simulink model "Final_EWASP_VC"  (R2022a)
settings: Solver=ode1  StartTime=0.0  StopTime=24*3600  FixedStep=10  RelTol=1e-3
values from neighbouring files (symbols this model uses):
  Aux_Threshold = 52    [Setup_Code_EWASP_VC.m]
  buildingAge = 2005    [Setup_Code_EWASP_VC.m]
  ceilingHeight = 2.4    [Setup_Code_EWASP_VC.m]
  conductiveHconnectMatrix = [ ... (first row only)    [Setup_Code_EWASP_VC.m]
  cRoofGreen = 100000    [Setup_Code_EWASP_VC.m]
  Defrost_After_Time = 30    [Setup_Code_EWASP_VC.m]
  DHWDemandProfile = occFreegainHotwaterElecTestPassiveOcc3(:,3)    [Setup_Code_EWASP_VC.m]
  Elec_Max = Elec_Max*(30/24.2)    [Setup_Code_EWASP_VC.m]
  Elec_Mid = Elec_Mid*(30/24.2)    [Setup_Code_EWASP_VC.m]
  Elec_Min = Elec_Min*(30/24.2)    [Setup_Code_EWASP_VC.m]
  ElecDemandProfile = occFreegainHotwaterElecTestPassiveOcc3(:,4)    [Setup_Code_EWASP_VC.m]
  ElecFixed = [Elec_Max(6,2) Elec_Max(6,4) Elec_Max(6,6) Elec_Max(6,7) ... (first row only)    [Setup_Code_EWASP_VC.m]
  floorOrCeilingArea = floorOrCeilingArea*1.15    [Setup_Code_EWASP_VC.m]
  forceCold = 0    [Setup_Code_EWASP_VC.m]
  freegain = occFreegainHotwaterElecTestPassiveOcc3(:,2)-max(occupancy)*25    [Setup_Code_EWASP_VC.m]
  furnitureModelOn = 1    [Setup_Code_EWASP_VC.m]
  Heat_Max = Heat_Max*(30/24.2)    [Setup_Code_EWASP_VC.m]
  Heat_Mid = Heat_Mid*(30/24.2)    [Setup_Code_EWASP_VC.m]
  Heat_Min = Heat_Min*(30/24.2)    [Setup_Code_EWASP_VC.m]
  HeatFixed = [Heat_Max(6,2) Heat_Max(6,4) Heat_Max(6,6) Heat_Max(6,7) ... (first row only)    [Setup_Code_EWASP_VC.m]
  HeatingOnProfile = repmat(HeatingOnProfile,365,1)    [Setup_Code_EWASP_VC.m]
  HEX_ReturnLowerLimit = 52.5    [Setup_Code_EWASP_VC.m]
  HEX_ReturnUpperLimit = 55    [Setup_Code_EWASP_VC.m]
  LeakMultiplier = 1+(2*(rand()-0.5)/10)    [Setup_Code_EWASP_VC.m]
  loopCap = 15    [Setup_Code_EWASP_VC.m]
  maxOcc = max(occupancyProfile)    [Setup_Code_EWASP_VC.m]
  NESW_wallArea = max(NESW_Lengths*ceilingHeight-NESW_Windows,0)    [Setup_Code_EWASP_VC.m]
  NESW_Windows = [ ... (first row only)    [Setup_Code_EWASP_VC.m]
  numRooms = roomCount    [Setup_Code_EWASP_VC.m]
  offsetDays = 0    [Setup_Code_EWASP_VC.m]
  pumpChoice = pumpChoices(MinIndex,1)    [Setup_Code_EWASP_VC.m]
  pumpRamp = 180    [Setup_Code_EWASP_VC.m]
  ReturnLowerLimit = 37.5    [Setup_Code_EWASP_VC.m]
  ReturnUpperLimit = 40    [Setup_Code_EWASP_VC.m]
  RoofIrradiance = Flat_NS_EW_RoofIrradiance(:,1)    [Setup_Code_EWASP_VC.m]
  roofStartTemp = ones(11,1)*20    [Setup_Code_EWASP_VC.m]
  rooftype = 0    [Setup_Code_EWASP_VC.m]
  RoomDataMatrix = [zeros(1,12);ones(1,12)*wallDensity;zeros(1,12);ones(1,12)*wallU;ones(1,12)*windowU;ones(1,12)*floorU;ones(1,12)*ceilingU;zeros(1,12);windowArea, 0;floorOrCeilingArea;zeros(1,12);floorOrCeilingArea*ceilingHeight]    [Setup_Code_EWASP_VC.m]
  roomVol = roomVol*1.15    [Setup_Code_EWASP_VC.m]
  slabStartTemp = (GroundTempTimeSeries(offsetDays*1440+1,1)+thermostatSetting)/2    [Setup_Code_EWASP_VC.m]
  SlackRequest = zeros(1440,1)    [Setup_Code_EWASP_VC.m]
  SolarThermalExists = 0    [Setup_Code_EWASP_VC.m]
  SourceFixed = HeatFixed-ElecFixed    [Setup_Code_EWASP_VC.m]
  StateSeries = StateSeriesGenerator(22,7,1)    [Setup_Code_EWASP_VC.m]
  Tank_Lower_Temp = 49.5    [Setup_Code_EWASP_VC.m]
  Tank_Upper_Temp = 52    [Setup_Code_EWASP_VC.m]
  Tank_Volume_m3 = 0.15    [Setup_Code_EWASP_VC.m]
  TankHeatHour = randi([1 5])-1    [Setup_Code_EWASP_VC.m]
  thermostatSetting = 20.0    (= 20)    [Setup_Code_EWASP_VC.m]
  upDown = [0;0;0;0;1;1;1;1;1;1;1]    [Setup_Code_EWASP_VC.m]
  variableASHP = 1    [Setup_Code_EWASP_VC.m]
  wallStartTempExt = thermostatSetting*(0.266+0.00215*outdoorStartTemp+0.018*wallU+0.00113*outdoorStartTemp*wallU+0.0068*wallU^2)    [Setup_Code_EWASP_VC.m]
undefined symbols (not defined in the file or in its folder): a, ceilingU, condUDMatrix, convUDMatrix, deltaPEXPANDED_E, deltaPEXPANDED_E2, deltaPEXPANDED_N, deltaPEXPANDED_N2, deltaPEXPANDED_S, deltaPEXPANDED_S2, deltaPEXPANDED_W, deltaPEXPANDED_W2, DesiredDHWTemp, DesiredFlowTempVsInOutDeltaTemp, DiffuseHorizontal, DiscIntNeverNeededParam, DNI, dwnAndConcrete, DWORK_A_HX, DWORK_CHK_FLU, DWORK_CP_NODE, DWORK_DH, DWORK_FLUID, DWORK_HCON, DWORK_LOSS, DWORK_MDOTDOWN, DWORK_MDOTIN, DWORK_MDOTUP, DWORK_MIX, DWORK_PRESS, DWORK_QDOTIN, DWORK_RHO_NODE, DWORK_TIN, DWORK_TS_OLD, DWORK_V_NODE, GroundTempTimeSeries, HCM, HCM2, HCM_closed, HCM_closed2, intermediateU, IsTop, massFlowMatrix, neighbourMatrix, numericalRoomUse, RadiatorMatrix, room2roomflowmatrix_E, room2roomflowmatrix_E2, room2roomflowmatrix_N, room2roomflowmatrix_N2, room2roomflowmatrix_S, room2roomflowmatrix_S2, room2roomflowmatrix_W, room2roomflowmatrix_W2, StateAirInEXPANDED_E, StateAirInEXPANDED_E2, StateAirInEXPANDED_N, StateAirInEXPANDED_N2, StateAirInEXPANDED_S, StateAirInEXPANDED_S2 ... (+23)
libraries: simulink x6, dspsigops x4, dspmtrx3 x4, carnot x3, spsEdgeDetectorLib x2, dspstat3 x2, powerlib_meascontrol x1, simulink_extras x1
(part 13 of 27)

== system Final_EWASP_VC/Airflow Model/Subsystem1/Subsystem ==
  In1 : Inport
  In2 : Inport  Port=2
  In3 : Inport  Port=3
  In4 : Inport  Port=4
  In5 : Inport  Port=5
  In6 : Inport  Port=6
  Abs{1..4,6} (5 alike) : Abs  SaturateOnIntegerOverflow=off
  Absolute Heat From : Product  Inputs=3
  Absolute Heat In2 : Product  Inputs=3
  Absolute Heat Out : Product  Inputs=3
  Absolute Heat Out1 : Product  Inputs=3
  Actual buoyancy : MATLAB Function  TreatAsAtomicUnit=on
  Add : Sum  Inputs=4
  Add1 : Sum  Inputs=4
  Add2 : Sum  Inputs=+-
  Air Heat capacity{,1..3} (4 alike) : Constant  Value=1000
  Celcius to Kelvin{,1,4..5} (4 alike) : Constant  Value=273.15
  "Determine flow in and flow out from net flow (+ve out, -ve in)" : Subsystem
  "Net flow out of room to neighbouring room (+ve out, -ve in)1" : Constant  Value=HCM_closed
  "Net flow out of room to neighbouring room (+ve out, -ve in)3" : Constant  Value=HCM
  "Net flow out of room to neighbouring room (+ve out, -ve in)5" : Constant  Value=VCM
  Product1 : Product
  Remove nan values : MATLAB Function  TreatAsAtomicUnit=on
  Saturation : Saturate  UpperLimit=100  LowerLimit=0
  Saturation1 : Saturate  UpperLimit=0  LowerLimit=-100
  Saturation2 : Saturate  UpperLimit=100  LowerLimit=0
  Saturation3 : Saturate  UpperLimit=0  LowerLimit=-100
  Subsystem : Subsystem
  Subsystem1 : Subsystem
      mask Display:
      | port_label('output', 1, 'Average_Density_Matrix')
      | port_label('output', 2, 'Delta_Density_Matrix')
      | port_label('input', 1, 'Room_Temp_Vector')
  Sum{,1,3..4} (4 alike) : Sum  Inputs=|++
  Sum of Elements : Sum  Inputs=+  CollapseMode=Specified dimension  CollapseDim=2
  Sum of Elements1 : Sum  Inputs=+  CollapseMode=Specified dimension  CollapseDim=2
  Sum2 : Sum  Inputs=+-
  Sum5 : Sum  Inputs=-++
  Sum6 : Sum  Inputs=+-
  max buoyancy : MATLAB Function  TreatAsAtomicUnit=on
  pflood : MATLAB Function  TreatAsAtomicUnit=on
  remove data no related to vertical flow : Constant  Value=VCM
  remove verical forced and closed door flow from bidirectinality calc1 : Product
  remove verical forced and closed door flow from bidirectinality calc2 : Product
  remove verical forced and closed door flow from bidirectinality calc : Product
  setnegative buoyancy flow to zero : Saturate  UpperLimit=100  LowerLimit=0
  tempVector to matrices : MATLAB Function  TreatAsAtomicUnit=on
  Out1 : Outport  VectorParamsAs1DForOutWhenUnconnected=off
  wires:
  [SAI] -> Absolute Heat In2/1
  [closed_out] -> Add1/2
  [open_out] -> Add1/1
  [R2R] -> remove verical forced and closed door flow from bidirectinality calc1/2, remove verical forced and closed door flow from bidirectinality calc/2
  remove data no related to vertical flow/1 -> Abs3/1
  "Net flow out of room to neighbouring room (+ve out, -ve in)1"/1 -> remove verical forced and closed door flow from bidirectinality calc1/1
  Sum1/1 -> Absolute Heat From/2
  Product1/1 -> Remove nan values/1(u)
  Saturation1/1 -> Abs1/1
  Abs3/1 -> Product1/2
  "Net flow out of room to neighbouring room (+ve out, -ve in)3"/1 -> remove verical forced and closed door flow from bidirectinality calc/1
  tempVector to matrices/1(y) -> [roomTempMatrix]
  setnegative buoyancy flow to zero/1 -> Product1/1
  remove verical forced and closed door flow from bidirectinality calc/1 -> "Determine flow in and flow out from net flow (+ve out, -ve in)"/1(In1)
  In6/1 -> [ODT]
  max buoyancy/1(y) -> Actual buoyancy/3(w)
  "Net flow out of room to neighbouring room (+ve out, -ve in)5"/1 -> Abs4/1
  Sum4/1 -> Absolute Heat In2/2
  Remove nan values/1(y) -> [buoyancy_in], [buoyancy_out]
  Sum of Elements1/1 -> Sum2/2
  Air Heat capacity/1 -> Absolute Heat Out/3
  Sum5/1 -> Out1/1
  Abs4/1 -> remove verical forced and closed door flow from bidirectinality calc2/2
  "Determine flow in and flow out from net flow (+ve out, -ve in)"/2(Out2) -> Subsystem/2(In2)
  remove verical forced and closed door flow from bidirectinality calc1/1 -> Saturation/1, Saturation1/1
  Add/1 -> Absolute Heat From/1, Add2/1
  Absolute Heat Out/1 -> Sum of Elements1/1
  Absolute Heat From/1 -> Sum of Elements/1
  Sum/1 -> Absolute Heat Out/2
  pflood/1(y) -> Abs2/1
  Saturation3/1 -> Abs6/1
  Abs6/1 -> [vforce_in]
  Saturation2/1 -> [vforce_out]
  Saturation/1 -> [closed_out]
  Add1/1 -> Add2/2, Absolute Heat Out/1
  Subsystem1/2(Out2) -> pflood/1(u)
  Absolute Heat In2/1 -> Sum5/3
  [TVT] -> Subsystem1/1(In1)
  remove verical forced and closed door flow from bidirectinality calc2/1 -> Saturation2/1, Saturation3/1
  [DP] -> Actual buoyancy/1(u)
  Sum2/1 -> Sum5/2
  [neighTempMatrix] -> Sum1/1
  [roomTempMatrix] -> Sum6/1
  Subsystem1/1(Out1) -> max buoyancy/1(u)
  Actual buoyancy/1(y) -> setnegative buoyancy flow to zero/1
  Abs2/1 -> Actual buoyancy/2(v), max buoyancy/2(v)
  [roomTempMatrix] -> Sum/1
  [SAO] -> Absolute Heat Out1/2
  Abs1/1 -> [closed_in]
  [neighTempMatrix] -> Sum6/2
  [R2R] -> remove verical forced and closed door flow from bidirectinality calc2/1
  Celcius to Kelvin5/1 -> Sum4/2
  Air Heat capacity3/1 -> Absolute Heat In2/3
  [TVT] -> tempVector to matrices/1(u)
  Celcius to Kelvin4/1 -> Sum3/2
  Air Heat capacity2/1 -> Absolute Heat Out1/3
  Celcius to Kelvin1/1 -> Sum1/2
  Air Heat capacity1/1 -> Absolute Heat From/3
  [TVT] -> Sum3/1
  tempVector to matrices/2(x) -> [neighTempMatrix]
  [ODT] -> Sum4/1
  In5/1 -> [TVT]
  Sum6/1 -> "Determine flow in and flow out from net flow (+ve out, -ve in)"/2(In2)
  [open_in] -> Add/1
  [closed_in] -> Add/2
  Celcius to Kelvin/1 -> Sum/2
  In2/1 -> [DP]
  In1/1 -> [R2R]
  In3/1 -> [SAO]
  In4/1 -> [SAI]
  Absolute Heat Out1/1 -> Sum5/1
  Sum3/1 -> Absolute Heat Out1/1
  Sum of Elements/1 -> Sum2/1
  "Determine flow in and flow out from net flow (+ve out, -ve in)"/1(Out1) -> Subsystem/1(In1)
  Subsystem/1(Out1) -> [open_in]
  Subsystem/2(Out2) -> [open_out]
  [vforce_in] -> Add/4
  [vforce_out] -> Add1/4
  [buoyancy_in] -> Add/3
  [buoyancy_out] -> Add1/3

== system Final_EWASP_VC/Airflow Model/Subsystem2/Subsystem ==
  In1 : Inport
  In2 : Inport  Port=2
  In3 : Inport  Port=3
  In4 : Inport  Port=4
  In5 : Inport  Port=5
  In6 : Inport  Port=6
  Abs{1..4,6} (5 alike) : Abs  SaturateOnIntegerOverflow=off
  Absolute Heat From : Product  Inputs=3
  Absolute Heat In2 : Product  Inputs=3
  Absolute Heat Out : Product  Inputs=3
  Absolute Heat Out1 : Product  Inputs=3
  Actual buoyancy : MATLAB Function  TreatAsAtomicUnit=on
  Add : Sum  Inputs=4
  Add1 : Sum  Inputs=4
  Air Heat capacity{,1..3} (4 alike) : Constant  Value=1000
  Celcius to Kelvin{,1,4..5} (4 alike) : Constant  Value=273.15
  "Determine flow in and flow out from net flow (+ve out, -ve in)" : Subsystem  TreatAsAtomicUnit=on
  "Net flow out of room to neighbouring room (+ve out, -ve in)1" : Constant  Value=HCM_closed2
  "Net flow out of room to neighbouring room (+ve out, -ve in)3" : Constant  Value=HCM2
  "Net flow out of room to neighbouring room (+ve out, -ve in)5" : Constant  Value=VCM2
  Product1 : Product
  Remove nan values : MATLAB Function  TreatAsAtomicUnit=on
  Saturation : Saturate  UpperLimit=100  LowerLimit=0
  Saturation1 : Saturate  UpperLimit=0  LowerLimit=-100
  Saturation2 : Saturate  UpperLimit=100  LowerLimit=0
  Saturation3 : Saturate  UpperLimit=0  LowerLimit=-100
  Subsystem1 : Subsystem
      mask Display:
      | port_label('output', 1, 'Average_Density_Matrix')
      | port_label('output', 2, 'Delta_Density_Matrix')
      | port_label('input', 1, 'Room_Temp_Vector')
  Sum{,1,3..4} (4 alike) : Sum  Inputs=|++
  Sum of Elements : Sum  Inputs=+  CollapseMode=Specified dimension  CollapseDim=2
  Sum of Elements1 : Sum  Inputs=+  CollapseMode=Specified dimension  CollapseDim=2
  Sum2 : Sum  Inputs=+-
  Sum5 : Sum  Inputs=-++
  Sum6 : Sum  Inputs=+-
  Sum7 : Sum  Inputs=|-+
  Symmetry Mod : Subsystem
  max buoyancy : MATLAB Function  TreatAsAtomicUnit=on
  pflood : MATLAB Function  TreatAsAtomicUnit=on
  remove data no related to vertical flow : Constant  Value=VCM2
  remove verical forced and closed door flow from bidirectinality calc1 : Product
  remove verical forced and closed door flow from bidirectinality calc2 : Product
  remove verical forced and closed door flow from bidirectinality calc : Product
  setnegative buoyancy flow to zero : Saturate  UpperLimit=100  LowerLimit=0
  tempVector to matrices : MATLAB Function  TreatAsAtomicUnit=on
  Out1 : Outport  VectorParamsAs1DForOutWhenUnconnected=off
  wires:
  [SAI] -> Absolute Heat In2/1
  [closed_out] -> Add1/2
  [open_out] -> Add1/1
  [R2R] -> remove verical forced and closed door flow from bidirectinality calc1/2, remove verical forced and closed door flow from bidirectinality calc/2
  remove data no related to vertical flow/1 -> Abs3/1
  "Net flow out of room to neighbouring room (+ve out, -ve in)1"/1 -> remove verical forced and closed door flow from bidirectinality calc1/1
  Sum1/1 -> Absolute Heat From/2
  Product1/1 -> Remove nan values/1(u)
  Saturation1/1 -> Abs1/1
  Abs3/1 -> Product1/2
  "Net flow out of room to neighbouring room (+ve out, -ve in)3"/1 -> remove verical forced and closed door flow from bidirectinality calc/1
  tempVector to matrices/1(y) -> [roomTempMatrix]
  setnegative buoyancy flow to zero/1 -> Product1/1
  remove verical forced and closed door flow from bidirectinality calc/1 -> "Determine flow in and flow out from net flow (+ve out, -ve in)"/1(In1)
  In6/1 -> [ODT]
  max buoyancy/1(y) -> Actual buoyancy/3(w)
  "Net flow out of room to neighbouring room (+ve out, -ve in)5"/1 -> Abs4/1
  Sum4/1 -> Absolute Heat In2/2
  Remove nan values/1(y) -> [buoyancy_in], [buoyancy_out]
  Air Heat capacity/1 -> Absolute Heat Out/3
  Sum5/1 -> Out1/1
  Abs4/1 -> remove verical forced and closed door flow from bidirectinality calc2/2
  remove verical forced and closed door flow from bidirectinality calc1/1 -> Saturation/1, Saturation1/1
  Sum/1 -> Absolute Heat Out/2
  pflood/1(y) -> Abs2/1
  [buoyancy_in] -> Add/3
  Saturation3/1 -> Abs6/1
  Abs6/1 -> [vforce_in]
  [vforce_out] -> Add1/4
  Saturation2/1 -> [vforce_out]
  Absolute Heat Out1/1 -> Sum7/1, Sum5/1
  Add1/1 -> Absolute Heat Out/1
  Subsystem1/2(Out2) -> pflood/1(u)
  Absolute Heat In2/1 -> Sum7/2, Sum5/3
  [TVT] -> Subsystem1/1(In1)
  remove verical forced and closed door flow from bidirectinality calc2/1 -> Saturation2/1, Saturation3/1
  "Determine flow in and flow out from net flow (+ve out, -ve in)"/1(Out1) -> Symmetry Mod/1(In1)
  [DP] -> Actual buoyancy/1(u)
  Sum2/1 -> Sum5/2
  [neighTempMatrix] -> Sum1/1
  [roomTempMatrix] -> Sum6/1
  Subsystem1/1(Out1) -> max buoyancy/1(u)
  Actual buoyancy/1(y) -> setnegative buoyancy flow to zero/1
  Abs2/1 -> Actual buoyancy/2(v), max buoyancy/2(v)
  [roomTempMatrix] -> Sum/1
  [SAO] -> Absolute Heat Out1/2
  [vforce_in] -> Add/4
  Abs1/1 -> [closed_in]
  [neighTempMatrix] -> Sum6/2
  [R2R] -> remove verical forced and closed door flow from bidirectinality calc2/1
  Celcius to Kelvin5/1 -> Sum4/2
  Air Heat capacity3/1 -> Absolute Heat In2/3
  [TVT] -> tempVector to matrices/1(u)
  Celcius to Kelvin4/1 -> Sum3/2
  Air Heat capacity2/1 -> Absolute Heat Out1/3
  Celcius to Kelvin1/1 -> Sum1/2
  Air Heat capacity1/1 -> Absolute Heat From/3
  [TVT] -> Sum3/1
  tempVector to matrices/2(x) -> [neighTempMatrix]
  Sum3/1 -> Absolute Heat Out1/1
  [ODT] -> Sum4/1
  In5/1 -> [TVT]
  Sum6/1 -> "Determine flow in and flow out from net flow (+ve out, -ve in)"/2(In2)
  [open_in] -> Add/1
  [closed_in] -> Add/2
  Celcius to Kelvin/1 -> Sum/2
  In2/1 -> [DP]
  In1/1 -> [R2R]
  In3/1 -> [SAO]
  In4/1 -> [SAI]
  Add/1 -> Absolute Heat From/1
  Sum of Elements/1 -> Sum2/1
  Sum of Elements1/1 -> Sum2/2
  Saturation/1 -> [closed_out]
  [buoyancy_out] -> Add1/3
  Absolute Heat From/1 -> Sum of Elements/1
  Absolute Heat Out/1 -> Sum of Elements1/1
  "Determine flow in and flow out from net flow (+ve out, -ve in)"/2(Out2) -> Symmetry Mod/2(In2)
  Symmetry Mod/1(Out1) -> [open_in]
  Symmetry Mod/2(Out2) -> [open_out]

== system Final_EWASP_VC/GSHP_Subsystem/DHW for GSHP case/HeatPump_Simplified ==
  THBsource : Inport
  THB_r : Inport  Port=2
  Tamb : Inport  Port=3
  Ctrl : Inport  Port=4
  mdot_cold : Inport  Port=5
  mdot_hot : Inport  Port=6
  HeatPump_basic : Subsystem  AncestorBlock=carnot/Basic/Thermal_Models/HeatPump_basic  mask(heat pump){K=K, caph=caph, capc=capc, UA=UA}
      mask prompts: K "Parameters K (see also HP_param.m)"; caph "thermal capacity hot loop [J/K]"; capc "thermal capacity cold loop [J/K]"; UA "heat loss coefficient [W/K]"
      mask help:
      | Linearized heat pump model, uses measured data according to EN 14511 as input (Schwamberger, K.: Fortschrittsberichete VDI, Nr. 263, 1991).
      | heating power: Qdot_h = K1*Tcold_in + K2*Thot_out + K3
      | electric power: Pel = K4*Tcold_in + K5*Thot_out + K6
      | source power: Qdot_c = -K7*Tcold_in - K8*Thot_out - K9
      | differential equation: cap*dTh/dt = Qdot + mdot*cp*(T_in-T) + UA*(Tamb-T)
      | with: cap = mass * heat_capactiy
      | See hp_param.m for the parameters K1 to K9.
      mask Help: web(fullfile(path_carnot('help'),'HeatPump_basic.html'),'-helpbrowser')
      mask DialogControl ParameterTabVar0 Prompt: HP Caracteristic
      mask DialogControl ParameterTabVar01 Prompt: Thermal
      mask Display: plot(0,-30,120,130,[30,46,36,46,36,46,30],[40,40,50,60,70,80,80],[70,54,64,54,64,54,64,54,64,54,70],[40,40,44,50,55,60,65,70,75,80,80],[56,45],[95,95],[51,51],[82,95])
  T_source : Outport  VectorParamsAs1DForOutWhenUnconnected=off
  "T_out " : Outport  Port=2  VectorParamsAs1DForOutWhenUnconnected=off
  HPdat : Outport  Port=3  VectorParamsAs1DForOutWhenUnconnected=off
  Real P_Therm : Outport  Port=4  VectorParamsAs1DForOutWhenUnconnected=off
  wires:
  HeatPump_basic/2(THBload) -> "T_out "/1  "THB_s"
  THBsource/1 -> HeatPump_basic/1(Tin_cold)
  THB_r/1 -> HeatPump_basic/2(Tin_hot)
  Tamb/1 -> HeatPump_basic/3(Tamb)
  Ctrl/1 -> HeatPump_basic/4(Ctrl)
  HeatPump_basic/1(Tsource) -> T_source/1  "THBsource"
  HeatPump_basic/3(HPdat) -> HPdat/1
  HeatPump_basic/4(Real P_Therm) -> Real P_Therm/1
  mdot_cold/1 -> HeatPump_basic/5(mdot_in_cold)
  mdot_hot/1 -> HeatPump_basic/6(mdot_in_hot)

== system Final_EWASP_VC/GSHP_Subsystem/DHW for GSHP case/Storage_Type_2_CONF ==
  note: upper heat exchanger (backup heater)
  note: pipe connection for DHW
  note: pipe connection for DHW circulation
  Tamb : Inport
  Temp_HX : Inport  Port=2
  THB_dhw : Inport  Port=3
  THB_circ : Inport  Port=4
  Mdot_dhw1 : Inport  Port=5
  Mdot_dhw2 : Inport  Port=6
  mdotHEX : Inport  Port=7
  HX_EN12977_1 : Subsystem  AncestorBlock=carnot/Storage/Thermal/Storage_Ports/HX_EN12977  mask(heat exchanger for storage, data EN 12977){h_in=hx1inlet, h_out=hx1outlet, hgt=hgt, dia=hx1dia, height=-0.68756, ua0=hx1uac, uam=hx1uam, uat=hx1uat, dpqua=hx1dpqua, nodes=nodes}
      mask prompts: h_in "relative height of inlet"; h_out "relative height of outlet"; hgt "Height of storage in m"; dia "Diameter of HX pipe [m]"; height "Height difference inlet-outlet [m]"; ua0 "uac: heat transfer coefficient [W/K /(kg/s) /(°C)]"; uam "uam: massflow dependent heat transfer [-]"; uat "uat: temperature difference dependent heat transfer [-]"; dpqua "Pressure drop coefficient dpqua [Pa/(kg/s)²]"; nodes "number of nodes"
      mask help:
      | The block transforms the incoming THV vector to a vector which the storage interprets as a heat exchanger.
      | Give inlet and outlet as a relative position 0=bottom to 1=top
      | The heat transfer is calculated by:
      | UA = uac * mdot^uam * ((Theatexchanger+Tstorage)/2)^uat
      mask init: same as Final_EWASP_VC/ASHP_Subsystem/DHW for ASHP Case/Storage_Type_2_CONF/HX_EN12977_1
      mask Help: web(['file:///' fullfile(path_carnot('help'),'StoragePorts_HeatExchangerModels.html')],'-helpbrowser')
      mask TypeOptions dia: Pressure_Drop_StorageHX/dia
      mask TypeOptions height: Pressure_Drop_StorageHX/hgt
      mask TypeOptions ua0: sfun_storage_heatexchanger/p1
      mask TypeOptions uam: sfun_storage_heatexchanger/p2
      mask TypeOptions uat: sfun_storage_heatexchanger/p3
      mask TypeOptions dpqua: Pressure_Drop_StorageHX/dpqua
      mask TypeOptions nodes: sfun_storage_heatexchanger/nodes
      mask DialogControl ParameterTabVar0 Prompt: Geometry
      mask DialogControl ParameterTabVar01 Prompt: Heat transfer
      mask DialogControl ParameterTabVar012 Prompt: Pressure drop
      mask DialogControl ParameterTabVar0123 Prompt: Calculation
      mask Display: disp('HX EN12977')
  Mux : Mux  Inputs=2
  Mux1 : Mux  Inputs=2
  Pipe_Connection_1 : Subsystem  AncestorBlock=carnot/Storage/Thermal/Storage_Ports/Pipe_Connection  mask(pipe connection to storage){h_in=pipe1inlet, h_out=pipe1outlet, hgt=hgt, nodes=nodes}
      mask prompts: h_in "relative height of inlet, range from 0 (= bottom) to 1 (= top)"; h_out "relative height of outlet, range from 0 (= bottom) to 1 (= top)"; hgt "Height of storage in m"; nodes "Number of nodes of storage (DO NOT CHANGE)"
      mask help: The block transforms the incoming THV vector to a vector which the storage interprets as a flow into the storage fluid.
      mask init: same as Final_EWASP_VC/ASHP_Subsystem/DHW for ASHP Case/Storage_Type_2_CONF/Pipe_Connection_1
      mask Help: web(fullfile(path_carnot('help'),'StoragePorts_PipeConnections.html'),'-helpbrowser')
      mask DialogControl ParameterTabVar0 Prompt: Geometry
      mask DialogControl ParameterTabVar02 Prompt: Calulation
      mask Display: disp('Pipe')
  Pipe_Connection_2 : Subsystem  AncestorBlock=carnot/Storage/Thermal/Storage_Ports/Pipe_Connection  mask(pipe connection to storage){h_in=pipe2inlet, h_out=pipe2outlet, hgt=hgt, nodes=nodes}
      mask prompts: h_in "relative height of inlet, range from 0 (= bottom) to 1 (= top)"; h_out "relative height of outlet, range from 0 (= bottom) to 1 (= top)"; hgt "Height of storage in m"; nodes "Number of nodes of storage (DO NOT CHANGE)"
      mask help: The block transforms the incoming THV vector to a vector which the storage interprets as a flow into the storage fluid.
      mask init: same as Final_EWASP_VC/ASHP_Subsystem/DHW for ASHP Case/Storage_Type_2_CONF/Pipe_Connection_1
      mask Help: web(fullfile(path_carnot('help'),'StoragePorts_PipeConnections.html'),'-helpbrowser')
      mask DialogControl ParameterTabVar0 Prompt: Geometry
      mask DialogControl ParameterTabVar02 Prompt: Calulation
      mask Display: disp('Pipe')
  Scope : Scope
  Scope1 : Scope
  Scope2 : Scope
  T_Sensor_Surface : carnot/Control/T_Sensor_Surface  pos=Tsensor  tdel=10  t0=mean(tini)
      settings: SourceProductName=Carnot
  Terminator1 : Terminator
  sfun_storageTnodesjh : S-Function  AncestorBlock=carnot/Basic/Thermal_Models/sfun_storageTnodes  FunctionName=storage_TnodesMOD  Parameters=dia, volume, standing, uloss , ubot, utop, cond, tini, nodes, nconnect, elimthermocline, condinvtc  SFunctionDeploymentMode=off  EnableBusSupport=off  SFcnStateName=DWORK_DH  mask(sfunction storage_Tnodes){uloss=uwall, ubot=ubot, utop=utop, cond=axcond, volume=volume, dia=dia, standing=standing cylinder, tini=tini, nodes=nodes, nconnect=3, elimthermocline=1, condinvtc=1e5}
      mask prompts: uloss "Heat transfer coefficient to ambient [W/m²K]"; ubot "Heat transfer coefficient to ambient bottom [W/m²K]"; utop "Heat transfer coefficient to ambient top [W/m²K]"; cond "Effective thermal conductivity [W/m/K]"; volume "Volume [m³]"; dia "Diameter [m]"; standing "Position"; tini "Initial temperature in °C"; nodes "Number of nodes"; nconnect "Number of ports"; elimthermocline "Elimination method (0 = off, 1 = temperature dependant, 2 = density dependant)"; condinvtc "COND_ITC: heat transport coefficient for the method 2"
      mask help:
      | The differential equation is derived from the energy conservation equation by using the finite volume method [Patankar: Numerical Heat Transfer and Fluid Flow, 1980].
      | Methods to eliminate the inversed thermocline (It occurs when node with lower density is below a node with higher density. Typically it can be translated to a node with higher temperature below a node with lower temperature. Exception is water below 4°C.):
      | 0 - inversed thermocline is not eliminated
      | 1 - Temperature based: An inversed thermocline exists , if the  temperature of the lower node is more than LIMIT_T_INVERSED degrees  above the upper node. In that case the temperatures of the nodes are mixed. For the geometry of a laying cylinder the different volumes of the nodes are taken in account.
      |  2 - Density based : An inversed thermocline exists, if the density of the lower node is less than the density of the upper node. The model  adds an additional heat transport towards the upper node:
      | heat transport [W/m³] = COND_ITC[W*m³/kg] * density_differnce[kg/m³] / node[m³]
      mask init: same as Final_EWASP_VC/ASHP_Subsystem/DHW for ASHP Case/Storage_Type_2_CONF/sfun_storageTnodesjh
      settings: SFcnIsStateOwnerBlock=on
      mask Help: web(fullfile(path_carnot('help'),'Storage_Type_N.html'),'-helpbrowser')
      mask TypeOptions standing: standing cylinder | lying cylinder
      mask DialogControl Container5 Prompt: Thermal
      mask DialogControl Container6 Prompt: Geometry
      mask DialogControl Container7 Prompt: Caclulation
      mask DialogControl Container10 Prompt: Inversed thermocline
      mask Display:
      | disp('storage_Tnodes')
      | 
      | port_label('input', 1, 'Tamb')
      | port_label('output', 1, 'Energy')
      | port_label('output', 2, 'Tnodes')
      | 
      | if exist('nconnect','var')
      |     for n = 1:nconnect
      |         port_label('input',  n+1, ['port' num2str(n)])
      |     end
      | end
  Tsensors : Outport  VectorParamsAs1DForOutWhenUnconnected=off
  THB_hx : Outport  Port=2  VectorParamsAs1DForOutWhenUnconnected=off
  THBdhw : Outport  Port=3  VectorParamsAs1DForOutWhenUnconnected=off
  AuxHeat : Outport  Port=4  VectorParamsAs1DForOutWhenUnconnected=off
  wires:
  HX_EN12977_1/1(to_storeT) -> sfun_storageTnodesjh/4
  Pipe_Connection_2/1(to_storeT) -> Scope/1, sfun_storageTnodesjh/3
  THB_circ/1 -> Mux1/1  "THBinPipe2"
  Tamb/1 -> sfun_storageTnodesjh/1  "Tamb"
  sfun_storageTnodesjh/2 -> Scope2/1, T_Sensor_Surface/1, HX_EN12977_1/1(from_storeT)  "Tnodes"
  Pipe_Connection_1/1(to_storeT) -> THBdhw/1, sfun_storageTnodesjh/2, Scope1/1
  Temp_HX/1 -> HX_EN12977_1/2(Tempin)
  HX_EN12977_1/2(TempHEXout) -> THB_hx/1
  T_Sensor_Surface/1 -> Tsensors/1
  Mdot_dhw1/1 -> Mux/2  "THBinPipe1"
  sfun_storageTnodesjh/1 -> Terminator1/1  "Energy"
  Mdot_dhw2/1 -> Mux1/2  "THBinPipe1"
  THB_dhw/1 -> Mux/1  "THBinPipe1"
  Mux/1 -> Pipe_Connection_1/1(THBin)
  Mux1/1 -> Pipe_Connection_2/1(THBin)
  mdotHEX/1 -> HX_EN12977_1/3(massFlowIn)
  HX_EN12977_1/3(AuxHeat) -> AuxHeat/1

== system Final_EWASP_VC/GSHP_Subsystem/DHW for GSHP case/Subsystem ==
  In1 : Inport
  Ceil : Rounding
  Clock : Clock
  Constant1 : Constant  Value=60
  Constant2 : Constant  Value=60
  Direct Lookup Table (n-D) : LookupNDDirect  NumberOfTableDimensions=1  TableIsInput=on
  Divide : Product  Inputs=*/
  Divide1 : Product  Inputs=*/
  Saturation : Saturate  UpperLimit=1440*365  LowerLimit=0
  Scope : Scope
  Out1 : Outport  VectorParamsAs1DForOutWhenUnconnected=off
  wires:
  Saturation/1 -> Scope/1, Direct Lookup Table (n-D)/1
  Divide1/1 -> Direct Lookup Table (n-D)/2
  Divide/1 -> Ceil/1
  Constant1/1 -> Divide/2
  In1/1 -> Divide1/1
  Direct Lookup Table (n-D)/1 -> Out1/1
  Constant2/1 -> Divide1/2
  Clock/1 -> Divide/1
  Ceil/1 -> Saturation/1

== system Final_EWASP_VC/GSHP_Subsystem/DHW for GSHP case/Switch Case Action Subsystem ==
  In1 : Inport
  Action Port : ActionPort  ActionPortLabel=default: { }
  1 m : Relay  OnSwitchValue=Tank_Upper_Temp  OffSwitchValue=Tank_Lower_Temp  OnOutputValue=0  OffOutputValue=1  OutDataTypeStr=boolean
  Out1 : Outport  VectorParamsAs1DForOutWhenUnconnected=off
  wires:
  In1/1 -> 1 m/1
  1 m/1 -> Out1/1

== system Final_EWASP_VC/GSHP_Subsystem/DHW for GSHP case/Switch Case Action Subsystem1 ==
  In1 : Inport
  Action Port : ActionPort  ActionPortLabel=case: { }
  'Aux Required' Alternative1 : Relay  OnSwitchValue=Aux_Threshold  OffSwitchValue=Aux_Threshold-0.1  OnOutputValue=0  OffOutputValue=1  OutDataTypeStr=boolean
  Out1 : Outport  VectorParamsAs1DForOutWhenUnconnected=off
  wires:
  In1/1 -> 'Aux Required' Alternative1/1
  'Aux Required' Alternative1/1 -> Out1/1

== system Final_EWASP_VC/GSHP_Subsystem/DHW for GSHP case/Switch Case Action Subsystem2 ==
  In1 : Inport
  Action Port : ActionPort  ActionPortLabel=default: { }
  1 means tank temp recently fell below 49.1 : Relay  OnSwitchValue=60  OffSwitchValue=49.5  OnOutputValue=0  OffOutputValue=1  OutDataTypeStr=boolean
  Out1 : Outport  VectorParamsAs1DForOutWhenUnconnected=off
  wires:
  In1/1 -> 1 means tank temp recently fell below 49.1/1
  1 means tank temp recently fell below 49.1/1 -> Out1/1

== system Final_EWASP_VC/GSHP_Subsystem/DHW for GSHP case/Switch Case Action Subsystem3 ==
  In1 : Inport
  Action Port : ActionPort  ActionPortLabel=case: { }
  'Aux Required' Alternative : Relay  OnSwitchValue=60  OffSwitchValue=Aux_Threshold  OnOutputValue=0  OffOutputValue=1  OutDataTypeStr=boolean
  Out1 : Outport  VectorParamsAs1DForOutWhenUnconnected=off
  wires:
  In1/1 -> 'Aux Required' Alternative/1
  'Aux Required' Alternative/1 -> Out1/1

== system Final_EWASP_VC/GSHP_Subsystem/Subsystem3/Ground_Source_Heat_Exchanger1 ==
  Tin : Inport
  Mdotin1 : Inport  Port=2
  Constant : Constant  Value=Ad
  Constant1 : Constant  Value=Au
  Constant10 : Constant  Value=Cd
  Constant11 : Constant  Value=Dd
  Constant12 : Constant  Value=Au0
  Constant13 : Constant  Value=Bu0
  Constant14 : Constant  Value=Cu
  Constant15 : Constant  Value=Du
  Constant2 : Constant  Value=Bd
  Constant3 : Constant  Value=Bu
  Constant4 : Constant  Value=Cd
  Constant5 : Constant  Value=Cu
  Constant6 : Constant  Value=Dd
  Constant7 : Constant  Value=Du
  Constant8 : Constant  Value=Ad0
  Constant9 : Constant  Value=Bd0
  Dd1 : Gain  Gain=Cdl  Multiplication=Matrix(K*u)  SaturateOnIntegerOverflow=on  OutDataTypeStr=Inherit: Same as input  ParamDataTypeStr=Inherit: Same as input
  Dd2 : Gain  Gain=c1  Multiplication=Matrix(K*u)  SaturateOnIntegerOverflow=on  OutDataTypeStr=Inherit: Same as input  ParamDataTypeStr=Inherit: Same as input
  Dd4 : Gain  Gain=Cdl  Multiplication=Matrix(K*u)  SaturateOnIntegerOverflow=on  OutDataTypeStr=Inherit: Same as input  ParamDataTypeStr=Inherit: Same as input
  Dd5 : Gain  Gain=c33  Multiplication=Matrix(K*u)  SaturateOnIntegerOverflow=on  OutDataTypeStr=Inherit: Same as input  ParamDataTypeStr=Inherit: Same as input
  Fcn : Fcn  Expr=u+273.15
  Fcn1 : Fcn  Expr=u-273.15
  Goto : Goto  TagVisibility=global
  K2C : Bias  Bias=-273.15  SaturateOnIntegerOverflow=off
  Mux1 : Mux  Inputs=2
  Mux2 : Mux  Inputs=2
  Mux4 : Mux  Inputs=2
  Randbedingung 1 : Subsystem
  Randbedingung 2 : Subsystem
  Sum : Sum  Inputs=|++  InputSameDT=on  SaturateOnIntegerOverflow=on  OutDataTypeStr=Inherit: Same as first input
  T_Earth : StateSpace  A=Ar  B=Br  C=Cr  D=Dr  InitialCondition=Tearth_anf(:)
  Tdown : Subsystem
  Tup : Subsystem
  mdot>0 : Subsystem
  mdot>1 : Subsystem
  mdot>2 : Subsystem
  mdot>3 : Subsystem
  mdot>4 : Subsystem
  mdot>5 : Subsystem
  mdot>6 : Subsystem
  mdot>7 : Subsystem
  out2d : Terminator
  out2u1 : Terminator
  out3d : Terminator
  out3u : Terminator
  parallel1 : Gain  Gain=1/np
  Tout : Outport  VectorParamsAs1DForOutWhenUnconnected=off
  Tnodes : Outport  Port=2  VectorParamsAs1DForOutWhenUnconnected=off
  tag scope: Au=global, B=global, Bu=global, C=global, Cu=global, D=global, Du=global
  wires:
  K2C/1 -> Tnodes/1
  Tin/1 -> Fcn/1
  Mdotin1/1 -> parallel1/1
  Mux1/1 -> K2C/1
  parallel1/1 -> mdot>7/2(mdot), mdot>6/2(mdot), mdot>5/2(mdot), mdot>4/2(mdot), mdot>3/2(mdot), mdot>2/2(mdot), mdot>1/2(mdot), mdot>0/2(mdot)
  Constant12/1 -> mdot>4/3(In4)
  Constant13/1 -> mdot>5/3(In4)
  Constant14/1 -> mdot>6/3(In4)
  Constant15/1 -> mdot>7/3(In4)
  mdot>4/1(Out1) -> [Au]
  mdot>5/1(Out1) -> [Bu]
  mdot>6/1(Out1) -> [Cu]
  mdot>7/1(Out1) -> [Du]
  Constant7/1 -> mdot>7/1(In1)
  Constant5/1 -> mdot>6/1(In1)
  Constant3/1 -> mdot>5/1(In1)
  Constant1/1 -> mdot>4/1(In1)
  Constant6/1 -> mdot>3/1(In1)
  Constant11/1 -> mdot>3/3(In4)
  Constant10/1 -> mdot>2/3(In4)
  mdot>3/1(Out1) -> [D]
  Constant4/1 -> mdot>2/1(In1)
  mdot>2/1(Out1) -> [C]
  Constant9/1 -> mdot>1/3(In4)
  Constant2/1 -> mdot>1/1(In1)
  Constant/1 -> mdot>0/1(In1)
  mdot>1/1(Out1) -> [B]
  Constant8/1 -> mdot>0/3(In4)
  mdot>0/1(Out1) -> Goto/1
  Tup/2(Out2) -> out2u1/1
  Tdown/2(Out2) -> out2d/1
  Tup/3(Out3) -> out3u/1
  Tdown/3(Out3) -> out3d/1
  Tdown/1(Out1) -> Randbedingung 1/2(T_Down), Dd1/1
  Mux2/1 -> Tdown/1(In1)
  Mux4/1 -> Tup/1(In1)
  Dd1/1 -> Mux4/1
  T_Earth/1 -> Mux1/1, Dd2/1  "T_Earth(i,j)"
  Tup/1(Out1) -> Randbedingung 1/1(T_Up), Dd4/1
  Dd4/1 -> Fcn1/1
  Dd5/1 -> Sum/1
  Randbedingung 2/1(T_Earth(i,DimRad) Gew) -> Sum/2
  Sum/1 -> T_Earth/1
  Randbedingung 1/1(T_Earth(i,0)) -> Dd5/1, Randbedingung 2/1(T_Earth(i,0))  "T_Earth(i,0)"
  Dd2/1 -> Mux4/2, Randbedingung 2/2(T_Earth(i,1)), Randbedingung 1/3(T_Earth(i,1)), Mux2/2  "T_Earth(i,1)"
  Randbedingung 2/2(T_Earth(i,DimRad)) -> Mux1/2
  Fcn1/1 -> Tout/1  "Tout"
  Fcn/1 -> Mux2/1

== system Final_EWASP_VC/GSHP_Subsystem/Subsystem3/HeatPump_Simplified ==
  THBsource : Inport
  THB_r : Inport  Port=2
  Tamb : Inport  Port=3
  Ctrl : Inport  Port=4
  mdot_cold : Inport  Port=5
  mdot_hot : Inport  Port=6
  power fraction : Inport  Port=7
  HeatPump_basic : Subsystem  AncestorBlock=carnot/Basic/Thermal_Models/HeatPump_basic  mask(heat pump){K=K, caph=caph, capc=capc, UA=UA}
      mask prompts: K "Parameters K (see also HP_param.m)"; caph "thermal capacity hot loop [J/K]"; capc "thermal capacity cold loop [J/K]"; UA "heat loss coefficient [W/K]"
      mask help:
      | Linearized heat pump model, uses measured data according to EN 14511 as input (Schwamberger, K.: Fortschrittsberichete VDI, Nr. 263, 1991).
      | heating power: Qdot_h = K1*Tcold_in + K2*Thot_out + K3
      | electric power: Pel = K4*Tcold_in + K5*Thot_out + K6
      | source power: Qdot_c = -K7*Tcold_in - K8*Thot_out - K9
      | differential equation: cap*dTh/dt = Qdot + mdot*cp*(T_in-T) + UA*(Tamb-T)
      | with: cap = mass * heat_capactiy
      | See hp_param.m for the parameters K1 to K9.
      mask Help: web(fullfile(path_carnot('help'),'HeatPump_basic.html'),'-helpbrowser')
      mask DialogControl ParameterTabVar0 Prompt: HP Caracteristic
      mask DialogControl ParameterTabVar01 Prompt: Thermal
      mask Display: plot(0,-30,120,130,[30,46,36,46,36,46,30],[40,40,50,60,70,80,80],[70,54,64,54,64,54,64,54,64,54,70],[40,40,44,50,55,60,65,70,75,80,80],[56,45],[95,95],[51,51],[82,95])
  T_source : Outport  VectorParamsAs1DForOutWhenUnconnected=off
  "T_out " : Outport  Port=2  VectorParamsAs1DForOutWhenUnconnected=off
  HPdat : Outport  Port=3  VectorParamsAs1DForOutWhenUnconnected=off
  Real P_Therm : Outport  Port=4  VectorParamsAs1DForOutWhenUnconnected=off
  wires:
  HeatPump_basic/2(THBload) -> "T_out "/1  "THB_s"
  THBsource/1 -> HeatPump_basic/1(Tin_cold)
  THB_r/1 -> HeatPump_basic/2(Tin_hot)
  Tamb/1 -> HeatPump_basic/3(Tamb)
  Ctrl/1 -> HeatPump_basic/4(Ctrl)
  HeatPump_basic/1(Tsource) -> T_source/1  "THBsource"
  HeatPump_basic/3(HPdat) -> HPdat/1
  HeatPump_basic/4(Real P_Therm) -> Real P_Therm/1
  mdot_cold/1 -> HeatPump_basic/5(mdot_in_cold)
  mdot_hot/1 -> HeatPump_basic/6(mdot_in_hot)
  power fraction/1 -> HeatPump_basic/7(Ctrl1)

== system Final_EWASP_VC/GSHP_Subsystem/Subsystem3/Instantaneous to kWh Total2 ==
  In1 : Inport
  Divide1 : Product  Inputs=*/
  Integrator23 : Integrator
  Tinitial9 : Constant  Value=3600000
  Out1 : Outport  VectorParamsAs1DForOutWhenUnconnected=off
  wires:
  Integrator23/1 -> Divide1/1
  Tinitial9/1 -> Divide1/2
  In1/1 -> Integrator23/1
  Divide1/1 -> Out1/1

== system Final_EWASP_VC/Subsystem_Room1/Lounge//Dining/Radiator w//Thermostatic Control2 ==
  In1 : Inport
  In3 : Inport  Port=2
  In2 : Inport  Port=3
  Add : Sum  Inputs=+-
  Constant : Constant  Value=Water_Volume
  Constant1 : Constant  Value=TRV_Therm_Setpoint
  Constant11 : Constant  Value=0
  Constant2 : Constant  Value=0.5
  Constant3 : Constant  Value=4180
  Constant6 : Constant  Value=40
  Constant7 : Constant  Value=40
  Discrete-Time Integrator : DiscreteIntegrator  InitialConditionSource=external  SampleTime=-1  ICPrevOutput=DiscIntNeverNeededParam  ICPrevScaledInput=DiscIntNeverNeededParam
  Discrete-Time Integrator1 : DiscreteIntegrator  InitialConditionSource=external  SampleTime=-1  ICPrevOutput=DiscIntNeverNeededParam  ICPrevScaledInput=DiscIntNeverNeededParam
  From : From
  Goto : Goto
  MATLAB Function : MATLAB Function  TreatAsAtomicUnit=on
  Product2 : Product
  Qdot2room1 : Scope
  Real-Imag to Complex : RealImagToComplex
  Saturation : Saturate  UpperLimit=1  LowerLimit=0
  Scope1 : Scope
  Sum2 : Sum
  const1 : Constant  Value=Power_Nominal
  dTnom : Constant  Value=DeltaT_Nominal
  Out3 : Outport  VectorParamsAs1DForOutWhenUnconnected=off
  Out1 : Outport  Port=2  VectorParamsAs1DForOutWhenUnconnected=off
  Out2 : Outport  Port=3  VectorParamsAs1DForOutWhenUnconnected=off
  wires:
  In1/1 -> MATLAB Function/9(Troom), Add/2
  In2/1 -> Product2/1
  Constant1/1 -> Add/1
  Add/1 -> Sum2/1
  Constant2/1 -> Sum2/2
  Sum2/1 -> Saturation/1
  Saturation/1 -> Qdot2room1/1, Product2/2
  Constant11/1 -> Real-Imag to Complex/2
  Discrete-Time Integrator/1 -> MATLAB Function/5(Tnode1)
  Real-Imag to Complex/1 -> MATLAB Function/8(nominalDeltaT)
  MATLAB Function/3(Qtoroom) -> Out3/1, Scope1/1
  Product2/1 -> MATLAB Function/3(mdotRad), Out2/1
  Constant3/1 -> MATLAB Function/2(heatCapRad)
  const1/1 -> MATLAB Function/7(nominalHeat)
  [B] -> Discrete-Time Integrator1/1
  Constant6/1 -> Discrete-Time Integrator/2
  dTnom/1 -> Real-Imag to Complex/1
  Constant7/1 -> Discrete-Time Integrator1/2
  MATLAB Function/1(deltaT1) -> Goto/1
  MATLAB Function/2(deltaT2) -> [B]
  Discrete-Time Integrator1/1 -> Out1/1, MATLAB Function/6(Tnode2)
  Constant/1 -> MATLAB Function/1(MassRad)
  In3/1 -> MATLAB Function/4(Tflow)
  From/1 -> Discrete-Time Integrator/1

== system Final_EWASP_VC/Subsystem_Room1/Lounge//Dining/Subsystem ==
  In1 : Inport
  In2 : Inport  Port=2
  In3 : Inport  Port=3
  In4 : Inport  Port=4
  In5 : Inport  Port=5
  In6 : Inport  Port=6
  In7 : Inport  Port=7
  Product : Product  Inputs=3
  Product1 : Product  Inputs=3
  Product2 : Product  Inputs=*/
  Sum : Sum  Inputs=+-
  Sum1 : Sum  Inputs=+-
  Sum2 : Sum
  Out1 : Outport  VectorParamsAs1DForOutWhenUnconnected=off
  wires:
  In6/1 -> Product1/3
  Sum/1 -> Product/1
  In1/1 -> Sum1/1, Sum/1
  In2/1 -> Sum/2
  In4/1 -> Product1/2, Product/2
  Sum1/1 -> Product1/1
  Product1/1 -> Sum2/2
  In5/1 -> Product/3
  In3/1 -> Sum1/2
  Product/1 -> Sum2/1
  Sum2/1 -> Product2/1
  In7/1 -> Product2/2
  Product2/1 -> Out1/1

== system Final_EWASP_VC/Subsystem_Room1/Lounge//Dining/Subsystem1 ==
  In1 : Inport
  In2 : Inport  Port=2
  In3 : Inport  Port=3
  In4 : Inport  Port=4
  In5 : Inport  Port=5
  Add : Sum
  Constant1 : Constant  Value=TemperatureSeries
  Constant2 : Constant  Value=offsetDays
  Constant3 : Constant  Value=0.3
  Constant4 : Constant  Value=offsetDays
  Digital Clock : DigitalClock  SampleTime=10
  Digital Clock1 : DigitalClock  SampleTime=10
  MATLAB Function : MATLAB Function  TreatAsAtomicUnit=on
  MATLAB Function1 : MATLAB Function  TreatAsAtomicUnit=on
  RoomNodeNumber1 : Constant  Value=wallHeatCapacityInt
  RoomNodeNumber2 : Constant  Value=Wall_Irradiance_Angles_NEWS
  RoomNodeNumber3 : Constant  Value=DNI
  RoomNodeNumber4 : Constant  Value=DiffuseHorizontal
  RoomNodeNumber5 : Constant  Value=NESW_wallArea
  RoomNodeNumber6 : Constant  Value=NESW_wallArea
  RoomNodeNumber7 : Constant  Value=wallHeatCapacityMid
  RoomNodeNumber8 : Constant  Value=wallHeatCapacityExt
  Scope : Scope
  Scope1 : Scope
  Scope2 : Scope  NumInputPorts=3
  Scope3 : Scope
  Terminator : Terminator
  Terminator1 : Terminator
  Windspeed : Constant  Value=windSpeedSeries
  integrate deltat's with initial wall temps as initial condition : Subsystem
  sum to give HEAT LOST (i.e. positive value is a loss) : Sum  Inputs=+
  uVal_Total for wall : Constant  Value=wallU
  Out1 : Outport  VectorParamsAs1DForOutWhenUnconnected=off
  Out2 : Outport  Port=2  VectorParamsAs1DForOutWhenUnconnected=off
  Out3 : Outport  Port=3  VectorParamsAs1DForOutWhenUnconnected=off
  Out4 : Outport  Port=4  VectorParamsAs1DForOutWhenUnconnected=off
  wires:
  Constant1/1 -> MATLAB Function/9(T_AmbientSeries)
  integrate deltat's with initial wall temps as initial condition/1(Out1) -> Scope2/1, MATLAB Function/5(T_InWallNEWS)
  RoomNodeNumber2/1 -> MATLAB Function1/1(angleSeries)
  RoomNodeNumber1/1 -> MATLAB Function/2(c_InPU)
  MATLAB Function/2(deltaTmid) -> Out3/1
  In5/1 -> MATLAB Function/8(T_Room)
  MATLAB Function1/2(NEWS_Irradiance) -> Terminator1/1
  MATLAB Function/4(logRoomHeatLoss) -> sum to give HEAT LOST (i.e. positive value is a loss)/1, Scope/1
  RoomNodeNumber8/1 -> MATLAB Function/4(c_OutPU), MATLAB Function1/9(c_OutPU)
  uVal_Total for wall/1 -> MATLAB Function/1(uValWall)
  In4/1 -> integrate deltat's with initial wall temps as initial condition/3(In3)
  Digital Clock/1 -> MATLAB Function1/4(Time)
  integrate deltat's with initial wall temps as initial condition/2(Out2) -> Scope2/2, Scope1/1, MATLAB Function/6(T_MidWallNEWS)
  RoomNodeNumber7/1 -> MATLAB Function/3(c_MidPU)
  RoomNodeNumber3/1 -> MATLAB Function1/2(DNISeries)
  integrate deltat's with initial wall temps as initial condition/3(Out3) -> Scope2/3, MATLAB Function/7(T_OutWallNEWS)
  MATLAB Function/1(deltaTint) -> Out2/1
  MATLAB Function/3(deltaTout) -> Add/2
  In3/1 -> integrate deltat's with initial wall temps as initial condition/2(In2)
  Windspeed/1 -> MATLAB Function/10(windSpeedSeries)
  Constant3/1 -> MATLAB Function1/6(SurfaceAlbedo)
  RoomNodeNumber4/1 -> MATLAB Function1/3(DiffSeries)
  In1/1 -> integrate deltat's with initial wall temps as initial condition/4(In4), Scope3/1, MATLAB Function/12(roomNumber), MATLAB Function1/8(roomNumber)
  MATLAB Function1/3(deltaTexternalNEWS) -> Add/1
  RoomNodeNumber5/1 -> MATLAB Function1/7(NESW_wallArea)
  RoomNodeNumber6/1 -> MATLAB Function/11(NESW_wallArea)
  Constant4/1 -> MATLAB Function/14(offsetDays)
  Constant2/1 -> MATLAB Function1/5(offsetDays)
  Digital Clock1/1 -> MATLAB Function/13(Time)
  MATLAB Function1/1(PU_AreaIrradianceTotal) -> Terminator/1
  In2/1 -> integrate deltat's with initial wall temps as initial condition/1(In1)
  sum to give HEAT LOST (i.e. positive value is a loss)/1 -> Out4/1
  Add/1 -> Out1/1

== system Final_EWASP_VC/Subsystem_Room1/Lounge//Dining/Subsystem2 ==
  In1 : Inport
  In2 : Inport  Port=2
  In3 : Inport  Port=3
  Constant1 : Constant  Value=[20;20;20;20]
  Constant2 : Constant  Value=offsetDays
  Constant3 : Constant  Value=90
  Constant4 : Constant  Value=[20;20;20;20]
  Digital Clock : DigitalClock  SampleTime=10
  Discrete-Time Integrator : DiscreteIntegrator  InitialConditionSource=external  SampleTime=-1  ICPrevOutput=DiscIntNeverNeededParam  ICPrevScaledInput=DiscIntNeverNeededParam
  Discrete-Time Integrator1 : DiscreteIntegrator  InitialConditionSource=external  SampleTime=-1  ICPrevOutput=DiscIntNeverNeededParam  ICPrevScaledInput=DiscIntNeverNeededParam
  Display : Display
  Display1 : Display
  Irradiance to Solar Gain1 : Subsystem
      mask Display:
      | port_label('input',1,'Incidence Angle')
      | port_label('input',2,'Tilt Angle')
      | port_label('input',3,'DNI')
      | port_label('input',4,'Diff_I')
      | port_label('output',1,'Qdot_SG')
      | port_label('output',2,'NEWS Absorbance')
      | disp('I2SG')
  MATLAB Function : MATLAB Function  TreatAsAtomicUnit=on
  MATLAB Function2 : MATLAB Function  TreatAsAtomicUnit=on
  RoomNodeNumber1 : Constant  Value=windowU
  RoomNodeNumber3 : Constant  Value=DNI
  RoomNodeNumber4 : Constant  Value=DiffuseHorizontal
  RoomNodeNumber5 : Constant  Value=NESW_Windows
  Sum of Elements : Sum  Inputs=+
  angle that DNI hits a NEWS wall/window as a function of time : Constant  Value=Wall_Irradiance_Angles_NEWS
  sum of heat GAINED by internal surfaces due to irradiance THROUGH window : Sum  Inputs=+
  Out1 : Outport  VectorParamsAs1DForOutWhenUnconnected=off
  Out2 : Outport  Port=2  VectorParamsAs1DForOutWhenUnconnected=off
  wires:
  Constant2/1 -> MATLAB Function2/5(offsetDays)
  MATLAB Function2/1(Angle_NEWS) -> Irradiance to Solar Gain1/1(In1)
  In1/1 -> MATLAB Function/8(roomNumber), MATLAB Function2/7(roomNumber)
  MATLAB Function2/2(NEWS_DNI) -> Irradiance to Solar Gain1/3(In3)
  angle that DNI hits a NEWS wall/window as a function of time/1 -> MATLAB Function2/1(angleSeries)
  sum of heat GAINED by internal surfaces due to irradiance THROUGH window/1 -> Out1/1
  Irradiance to Solar Gain1/1(Out1) -> sum of heat GAINED by internal surfaces due to irradiance THROUGH window/1
  Digital Clock/1 -> MATLAB Function2/4(Time)
  RoomNodeNumber3/1 -> MATLAB Function2/2(DNISeries)
  RoomNodeNumber4/1 -> MATLAB Function2/3(DiffSeries)
  Constant3/1 -> Irradiance to Solar Gain1/2(In2)
  RoomNodeNumber5/1 -> MATLAB Function/3(NESW_Windows), MATLAB Function2/6(NESW_Windows)
  MATLAB Function2/3(NEWS_Diff) -> Irradiance to Solar Gain1/4(In4)
  Irradiance to Solar Gain1/2(Out2) -> MATLAB Function/6(absorbedNEWS)
  In2/1 -> [Tin]
  In3/1 -> [Tout]
  [Tout] -> MATLAB Function/5(outdoorTemp)
  [Tin] -> MATLAB Function/4(roomTemp)
  RoomNodeNumber1/1 -> MATLAB Function/7(windowUval)
  [deltaT_window_In] -> Discrete-Time Integrator/1
  [deltaT_window_Out] -> Discrete-Time Integrator1/1
  Constant1/1 -> Discrete-Time Integrator/2
  Constant4/1 -> Discrete-Time Integrator1/2
  Discrete-Time Integrator/1 -> Display1/1, MATLAB Function/1(windowTempsNEWS_in)
  Discrete-Time Integrator1/1 -> MATLAB Function/2(windowTempsNEWS_out)
  MATLAB Function/1(deltaT_win_in) -> [deltaT_window_In]
  MATLAB Function/2(deltaT_win_out) -> [deltaT_window_Out]
  MATLAB Function/3(Q_to_room) -> Sum of Elements/1, Display/1
  Sum of Elements/1 -> Out2/1
